simulink model "ETC"  (R2020a)
settings: Solver=VariableStepAuto  StartTime=0.0  StopTime=20  RelTol=1e-3
model workspace (MAT data in the model file):
  J = Simulink.Parameter
  J.Value = 0.004
  J.DataType = 'auto'
  J.Dimensions = [1 1]
  Km = Simulink.Parameter
  Km.Value = 0.0186
  Km.DataType = 'auto'
  Km.Dimensions = [1 1]
  Ks = Simulink.Parameter
  Ks.Value = 0.1213
  Ks.DataType = 'auto'
  Ks.Dimensions = [1 1]
  R = Simulink.Parameter
  R.Value = 2.263
  R.DataType = 'auto'
  R.Dimensions = [1 1]
  n = Simulink.Parameter
  n.Value = 20
  n.DataType = 'auto'
  n.Dimensions = [1 1]
settings Model: OrderedModelArguments=off  Creator=44689  LastModifiedBy=44689

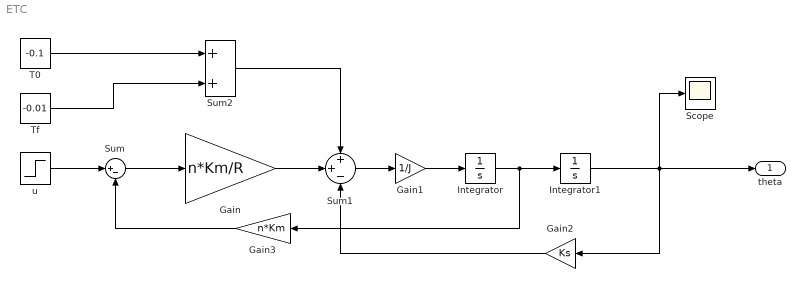
== system ETC ==
  Gain : Gain  Gain=n*Km/R
  Gain1 : Gain  Gain=1/J
  Gain2 : Gain  Gain=Ks
  Gain3 : Gain  Gain=n*Km
  Integrator : Integrator
  Integrator1 : Integrator
  Scope : Scope
  Sum : Sum  Inputs=|+-
  Sum1 : Sum  Inputs=++-
  Sum2 : Sum
  T0 : Constant  Value=-0.1
  Tf : Constant  Value=-0.01
  u : Step  Time=10  Before=8  After=13.8  SampleTime=0
  theta : Outport
  wires:
  Integrator/1 -> Integrator1/1, Gain3/1
  u/1 -> Sum/1
  Sum/1 -> Gain/1
  Gain1/1 -> Integrator/1
  Gain/1 -> Sum1/2
  Sum1/1 -> Gain1/1
  T0/1 -> Sum2/1
  Tf/1 -> Sum2/2
  Sum2/1 -> Sum1/1
  Gain2/1 -> Sum1/3
  Gain3/1 -> Sum/2
  Integrator1/1 -> Scope/1, Gain2/1, theta/1
